simulink model "chap5_10sim"  (Simulink 7.7)
settings: Solver=ode45  StartTime=0.0  StopTime=10  FixedStep=0.001  RelTol=1e-3
settings Model: Creator=hp  LastModifiedBy=ljk
settings OptimizationCC: InitFltsAndDblsToZero=on
settings DebuggingCC: SaveWithParameterizedLinksMsg=none  SignalResolutionControl=TryResolveAllWithWarning  SolverPrmCheckMsg=none  MultiTaskDSMMsg=warning  MultiTaskCondExecSysMsg=none  StrictBusMsg=Warning
settings RTWCC: IncludeERTFirstTime=on
settings GRTTargetCC: TargetFcnLib=ansi_tfl_tmw.mat

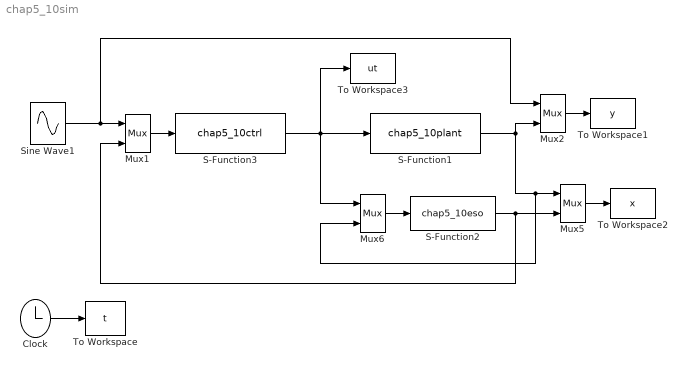
== system chap5_10sim ==
  Clock : Clock
      settings: Decimation=30
  Mux{1..2,5..6} (4 alike) : Mux  Inputs=2
  S-Function1 : S-Function  FunctionName=chap5_10plant  EnableBusSupport=off
  S-Function2 : S-Function  FunctionName=chap5_10eso  EnableBusSupport=off
  S-Function3 : S-Function  FunctionName=chap5_10ctrl  EnableBusSupport=off
  Sine Wave1 : Sin  SampleTime=0
  To Workspace : ToWorkspace  VariableName=t  SampleTime=-1  SaveFormat=Array
  To Workspace1 : ToWorkspace  VariableName=y  SampleTime=-1  SaveFormat=Array
  To Workspace2 : ToWorkspace  VariableName=x  SampleTime=-1  SaveFormat=Array
  To Workspace3 : ToWorkspace  VariableName=ut  SampleTime=-1  SaveFormat=Array
  wires:
  Mux6/1 -> S-Function2/1
  Clock/1 -> To Workspace/1
  S-Function1/1 -> Mux5/1, Mux6/2, Mux2/2
  S-Function2/1 -> Mux5/2, Mux1/2
  Mux5/1 -> To Workspace2/1
  Sine Wave1/1 -> Mux1/1, Mux2/1
  Mux1/1 -> S-Function3/1
  S-Function3/1 -> S-Function1/1, To Workspace3/1, Mux6/1
  Mux2/1 -> To Workspace1/1
